simulink model "Flight_mechanics"  (R2025b)
settings: Solver=ode4  StartTime=0.0  StopTime=50  FixedStep=0.01  RelTol=1e-3
undefined symbols (not defined in the file): a_coef_body, m_mass
libraries: aerolibadyn x1
settings Model: DataDictionary=Aerodynamic_data.sldd  Creator=mauro  LastModifiedBy=mauro

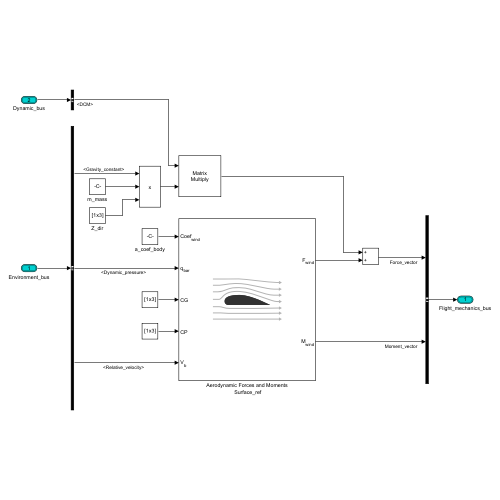
[thumbnail: Simulink's stored preview of the top-level diagram]
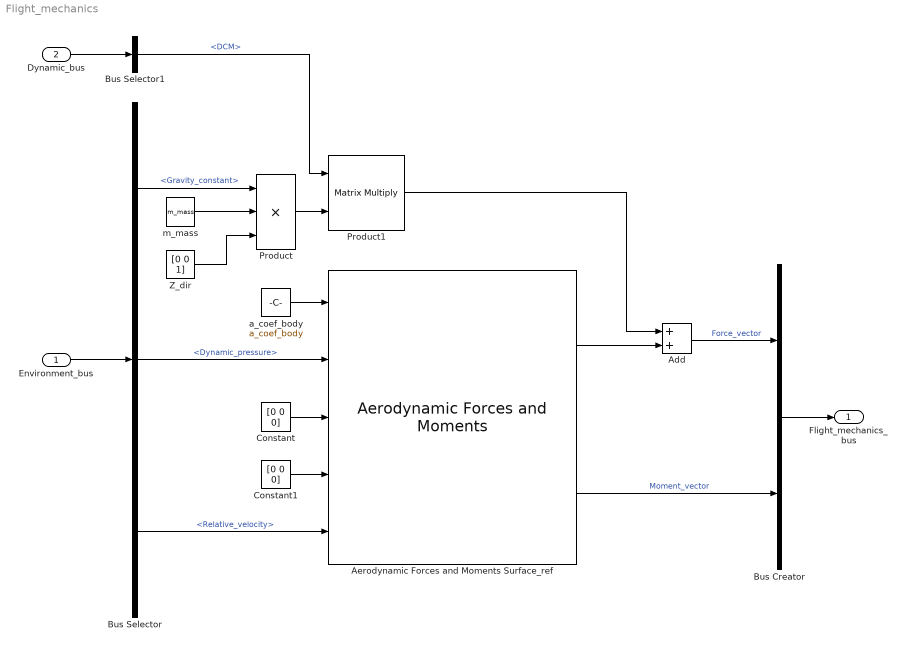
== system Flight_mechanics ==
  Environment_bus : Inport  OutDataTypeStr=Bus: Environment_bus  BusOutputAsStruct=on
  Dynamic_bus : Inport  Port=2  OutDataTypeStr=Bus: Dynamic_bus  BusOutputAsStruct=on
  Add : Sum
  Aerodynamic Forces and Moments Surface_ref : aerolibadyn/Aerodynamic Forces and Moments   inputAxes=Wind  outputForceAxes=Wind  outputMomentAxes=Wind  S=a_surface_ref  b=0  cbar=0
  Bus Creator : BusCreator  Inputs=2  OutDataTypeStr=Bus: Flight_mechanics_bus  NonVirtualBus=on
  Bus Selector : BusSelector  OutputSignals=Gravity_constant,Dynamic_pressure,Relative_velocity
  Bus Selector1 : BusSelector  OutputSignals=DCM
  Constant : Constant  Value=[0 0 0]
  Constant1 : Constant  Value=[0 0 0]
  Product : Product  Inputs=3
  Product1 : Product  Multiplication=Matrix(*)
  Z_dir : Constant  Value=[0 0 1]
  a_coef_body : Constant  Value=a_coef_body
  m_mass : Constant  Value=m_mass
  Flight_mechanics_bus : Outport  OutDataTypeStr=Bus: Flight_mechanics_bus  BusOutputAsStruct=on
  wires:
  a_coef_body/1 -> Aerodynamic Forces and Moments Surface_ref/1
  Environment_bus/1 -> Bus Selector/1
  Bus Selector/2 -> Aerodynamic Forces and Moments Surface_ref/2  "<Dynamic_pressure>"
  m_mass/1 -> Product/2
  Aerodynamic Forces and Moments Surface_ref/1 -> Add/2
  Aerodynamic Forces and Moments Surface_ref/2 -> Bus Creator/2  "Moment_vector"
  Add/1 -> Bus Creator/1  "Force_vector"
  Bus Creator/1 -> Flight_mechanics_bus/1
  Product1/1 -> Add/1
  Product/1 -> Product1/2
  Bus Selector/3 -> Aerodynamic Forces and Moments Surface_ref/5  "<Relative_velocity>"
  Dynamic_bus/1 -> Bus Selector1/1
  Bus Selector1/1 -> Product1/1  "<DCM>"
  Z_dir/1 -> Product/3
  Bus Selector/1 -> Product/1  "<Gravity_constant>"
  Constant/1 -> Aerodynamic Forces and Moments Surface_ref/3
  Constant1/1 -> Aerodynamic Forces and Moments Surface_ref/4
